simulink model "ques6"  (R2020a)
settings: Solver=VariableStepAuto  StartTime=0.0  StopTime=10.0  RelTol=1e-3
libraries: simulink x1
settings Model: Creator=kiran  LastModifiedBy=kiran

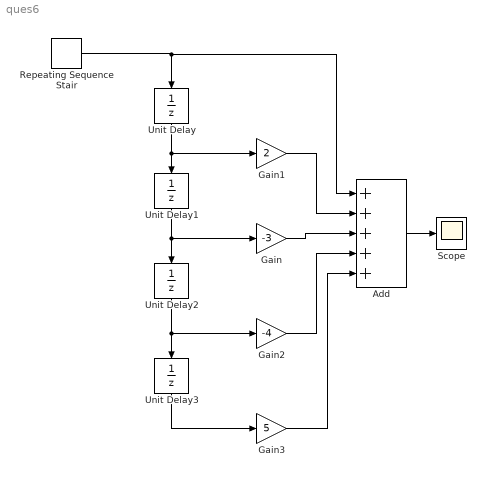
== system ques6 ==
  Add : Sum  Inputs=+++++
  Gain : Gain  Gain=-3
  Gain1 : Gain  Gain=2
  Gain2 : Gain  Gain=-4
  Gain3 : Gain  Gain=5
  Repeating Sequence Stair : simulink/Sources/Repeating Sequence Stair  OutValues=[3 1 4 2 1].'  tsamp=-1  OutMin=[]  OutMax=[]  OutDataTypeStr=double  OutputDataTypeScalingMode=double  OutDataType=fixdt(0,8)  ConRadixGroup=Best Precision: Vector-wise  OutScaling=2^-12
  Scope : Scope
  Unit Delay{,1..3} (4 alike) : UnitDelay  SampleTime=-1  HasFrameUpgradeWarning=on
  wires:
  Add/1 -> Scope/1
  Gain1/1 -> Add/2
  Gain/1 -> Add/3
  Gain2/1 -> Add/4
  Gain3/1 -> Add/5
  Repeating Sequence Stair/1 -> Add/1, Unit Delay/1
  Unit Delay/1 -> Unit Delay1/1, Gain1/1
  Unit Delay1/1 -> Unit Delay2/1, Gain/1
  Unit Delay2/1 -> Gain2/1, Unit Delay3/1
  Unit Delay3/1 -> Gain3/1
